simulink model "ofdm_isi"  (R2021a)
settings: Solver=FixedStepDiscrete  StartTime=0.0  StopTime=1e-2  FixedStep=25e-9  RelTol=1e-3
undefined symbols (not defined in the file): Radix
libraries: simulink x5, dspxfrm3 x2, commchan3 x1, commrandsrc2 x1, dspswit3 x1, commsink2 x1, commofdm x1
settings Model: Creator=Administrator  LastModifiedBy=Administrator

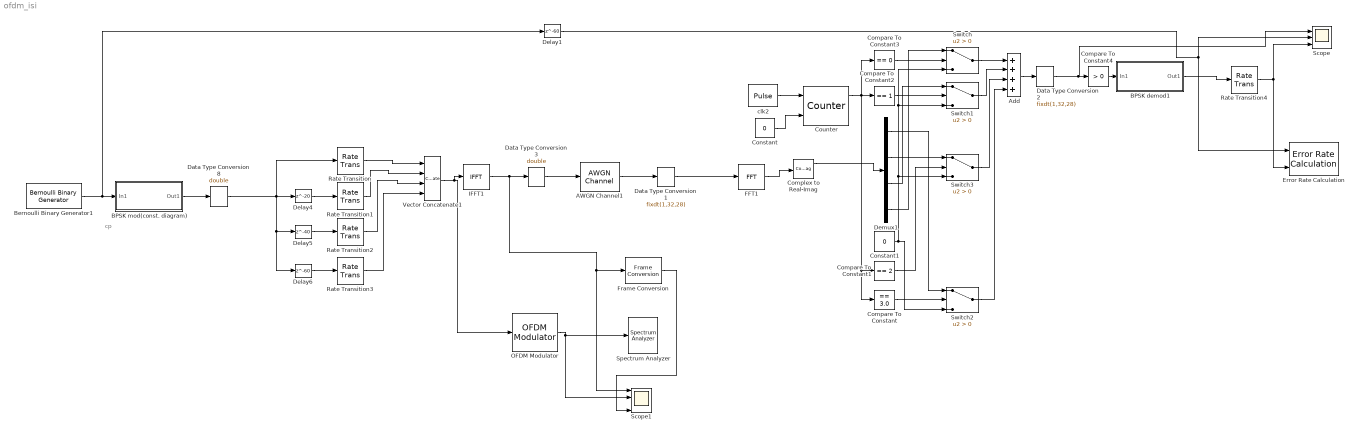
== system ofdm_isi ==
  note: cp
  AWGN Channel1 : commchan3/AWGN Channel  InputProcessing=Columns as channels (frame based)  seed=23  noiseMode="Signal to noise ratio  (Eb/No)"  EbNodB=25  EsNodB=10  SNRdB=10  bitsPerSym=1  Ps=1  Tsym=1/2e6  variance=1
  Add : Sum  Inputs=++++
  BPSK demod1 : Subsystem
  BPSK mod(const. diagram) : Subsystem
  Bernoulli Binary Generator1 : commrandsrc2/Bernoulli Binary Generator  P=0.3  seed=43  Ts=1/2e6  frameBased=off  sampPerFrame=1  orient=off  outDataType=double
      settings: SourceProductBaseCode=CM
  Compare To Constant : simulink/Logic and Bit Operations/Compare To Constant  relop===  const=3.0  OutDataTypeStr=boolean
  Compare To Constant1 : simulink/Logic and Bit Operations/Compare To Constant  relop===  const=2  OutDataTypeStr=boolean
  Compare To Constant2 : simulink/Logic and Bit Operations/Compare To Constant  relop===  const=1  OutDataTypeStr=boolean
  Compare To Constant3 : simulink/Logic and Bit Operations/Compare To Constant  relop===  const=0  OutDataTypeStr=boolean
  Compare To Constant4 : simulink/Logic and Bit Operations/Compare To Constant  relop=>  const=0  OutDataTypeStr=boolean
  Complex to Real-Imag : ComplexToRealImag
  Constant : Constant  Value=0  SampleTime=25e-9
  Constant1 : Constant  Value=0
  Counter : dspswit3/Counter  Direction=Up  CountEvent=Rising edge  CounterSize=User defined  MaxCount=3  InitialCount=0  Output=Count and Hit  HitValue=3  ResetInput=on  SamplesPerFrame=1  Ts=1  CntDtype=double  HitDtype=Logical
  Data Type Conversion1 : DataTypeConversion  OutMax=[1]  OutDataTypeStr=fixdt(1,32,28)  RndMeth=Nearest
  Data Type Conversion2 : DataTypeConversion  OutMax=[1]  OutDataTypeStr=fixdt(1,32,28)  RndMeth=Nearest
  Data Type Conversion3 : DataTypeConversion  OutMax=[1]  OutDataTypeStr=double  RndMeth=Nearest
  Data Type Conversion8 : DataTypeConversion  OutMax=[1]  OutDataTypeStr=double  RndMeth=Nearest
  Delay1 : Delay  DelayLength=60  SampleTime=25e-9
  Delay4 : Delay  DelayLength=20  SampleTime=25e-9
  Delay5 : Delay  DelayLength=40  SampleTime=25e-9
  Delay6 : Delay  DelayLength=60  SampleTime=25e-9
  Demux1 : Demux
      settings: DisplayOption=none
  Error Rate Calculation : commsink2/Error Rate Calculation  N=0  st_delay=0  cp_mode=Entire frame  subframe=[]  PMode=Workspace  WsName=OFDM_1  RsMode2=off  stop=off  numErr=100  maxBits=1e6
  FFT1 : dspxfrm3/FFT  FFTImplementation=Radix-2  CompMethod=Table lookup  TableOpt=NEW  TableOptActive=Speed  BitRevOrder=off  Normalize=on  InheritFFTLength=on  FFTLength=4  WrapInput=on  roundingMode=Floor  overflowMode=off  firstCoeffMode=Specify word length  firstCoeffWordLength=32  firstCoeffFracLength=15  firstCoeffDataTypeStr=fixdt(1,32)  firstCoeffLastDataTypeStr=fixdt(1,32)  prodOutputMode=Binary point scaling  prodOutputWordLength=32  prodOutputFracLength=28  prodOutputDataTypeStr=fixdt(1,32,28)  prodOutputLastDataTypeStr=fixdt(1,32,28)  accumMode=Binary point scaling  accumWordLength=32  accumFracLength=28  accumDataTypeStr=fixdt(1,32,28)  accumLastDataTypeStr=fixdt(1,32,28)  outputMode=Binary point scaling  outputWordLength=32  outputFracLength=28  outputDataTypeStr=fixdt(1,32,28)  outputMin=[]  outputMax=[]  outputLastDataTypeStr=fixdt(1,32,28)
  Frame Conversion : FrameConversion  OutFrame=Sample-based
  IFFT1 : dspxfrm3/IFFT  FFTImplementation=Radix-2  CompMethod=Table lookup  TableOpt=NEW  TableOptActive=Speed  BitRevOrder=off  cs_in=off  Normalize=off  InheritFFTLength=off  FFTLength=4  WrapInput=on  mode=Complex  outSamplingMode=Sample based  roundingMode=Floor  overflowMode=off  firstCoeffMode=Specify word length  firstCoeffWordLength=32  firstCoeffFracLength=15  firstCoeffDataTypeStr=fixdt(1,32)  firstCoeffLastDataTypeStr=fixdt(1,32)  prodOutputMode=Binary point scaling  prodOutputWordLength=32  prodOutputFracLength=28  prodOutputDataTypeStr=fixdt(1,32,28)  prodOutputLastDataTypeStr=fixdt(1,32,28)  accumMode=Binary point scaling  accumWordLength=32  accumFracLength=28  accumDataTypeStr=fixdt(1,32,28)  accumLastDataTypeStr=fixdt(1,32,28)  outputMode=Binary point scaling  outputWordLength=32  outputFracLength=28  outputDataTypeStr=fixdt(1,32,28)  outputMin=[]  outputMax=[]  outputLastDataTypeStr=fixdt(1,32,28)
  OFDM Modulator : commofdm/OFDM Modulator  StatePerturbationForJacobian=1.0e-05  FFTLength=9  NumGuardBandCarriers=[3; 2]  InsertDCNull=off  PilotInputPort=off  PilotCarrierIndices=[12; 26; 40; 54]  CyclicPrefixLength=2  Windowing=off  WindowLength=1  NumSymbols=1  NumTransmitAntennas=1  SimulateUsing=Code generation
      settings: SourceProductBaseCode=CM
  Rate Transition{,1..3} (4 alike) : RateTransition  OutPortSampleTimeMultiple=1/3  OutPortSampleTime=4/2e6
  Rate Transition4 : RateTransition  OutPortSampleTimeMultiple=1/3  OutPortSampleTime=1/2e6
  Scope : Scope  NumInputPorts=3
  Scope1 : Scope  NumInputPorts=4
  Spectrum Analyzer : SpectrumAnalyzer
  Switch{,1..3} (4 alike) : Switch  Criteria=u2 > Threshold
  Vector Concatenate1 : Concatenate  NumInputs=4
  clk2 : DiscretePulseGenerator  PulseType=Time based  Period=1/2e6  PulseWidth=50
  wires:
  Switch2/1 -> Add/4
  Demux1/3 -> Switch1/1
  Rate Transition/1 -> Vector Concatenate1/1
  Delay1/1 -> Error Rate Calculation/1, Scope/2
  Rate Transition4/1 -> Error Rate Calculation/2, Scope/3
  Compare To Constant4/1 -> BPSK demod1/1(In1)
  Switch1/1 -> Add/2
  FFT1/1 -> Complex to Real-Imag/1
  Rate Transition3/1 -> Vector Concatenate1/4
  Rate Transition2/1 -> Vector Concatenate1/3
  clk2/1 -> Counter/1
  Complex to Real-Imag/1 -> Demux1/1
  Add/1 -> Data Type Conversion2/1
  Constant/1 -> Counter/2
  Counter/1 -> Compare To Constant1/1, Compare To Constant/1, Compare To Constant2/1, Compare To Constant3/1
  Compare To Constant1/1 -> Switch3/2
  AWGN Channel1/1 -> Data Type Conversion1/1
  Demux1/1 -> Switch2/1
  BPSK mod(const. diagram)/1(Out1) -> Data Type Conversion8/1
  Demux1/4 -> Switch/1
  Switch/1 -> Add/1
  Bernoulli Binary Generator1/1 -> BPSK mod(const. diagram)/1(In1), Delay1/1
  IFFT1/1 -> Scope1/1, Frame Conversion/1, Data Type Conversion3/1
  BPSK demod1/1(Out1) -> Rate Transition4/1
  Constant1/1 -> Switch1/3, Switch/3, Switch3/3, Switch2/3
  Compare To Constant/1 -> Switch2/2
  Delay6/1 -> Rate Transition3/1
  Demux1/2 -> Switch3/1
  Delay4/1 -> Rate Transition1/1
  Compare To Constant2/1 -> Switch1/2
  Rate Transition1/1 -> Vector Concatenate1/2
  Switch3/1 -> Add/3
  Delay5/1 -> Rate Transition2/1
  Compare To Constant3/1 -> Switch/2
  Data Type Conversion8/1 -> Rate Transition/1, Delay6/1, Delay5/1, Delay4/1
  Data Type Conversion1/1 -> FFT1/1
  Data Type Conversion2/1 -> Scope/1, Compare To Constant4/1
  Data Type Conversion3/1 -> AWGN Channel1/1
  OFDM Modulator/1 -> Scope1/2, Spectrum Analyzer/1
  Vector Concatenate1/1 -> IFFT1/1, OFDM Modulator/1
  Frame Conversion/1 -> Scope1/4

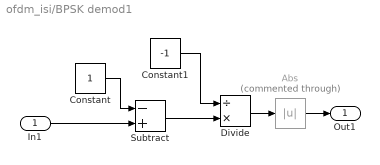
== system ofdm_isi/BPSK demod1 ==
  In1 : Inport
  Abs : Abs  Commented=through
  Constant : Constant
  Constant1 : Constant  Value=-1
  Divide : Product  Inputs=/*
  Subtract : Sum  Inputs=-+
  Out1 : Outport
  wires:
  Constant/1 -> Subtract/1
  Subtract/1 -> Divide/2
  Constant1/1 -> Divide/1
  In1/1 -> Subtract/2
  Divide/1 -> Abs/1
  Abs/1 -> Out1/1

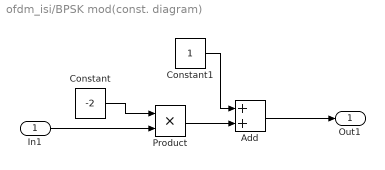
== system ofdm_isi/BPSK mod(const. diagram) ==
  In1 : Inport
  Add : Sum
  Constant : Constant  Value=-2
  Constant1 : Constant
  Product : Product
  Out1 : Outport
  wires:
  Constant/1 -> Product/1
  In1/1 -> Product/2
  Product/1 -> Add/2
  Constant1/1 -> Add/1
  Add/1 -> Out1/1
